simulink model "Target_Control_System"  (R2021b)
settings: Solver=FixedStepDiscrete  StartTime=0.0  StopTime=5  RelTol=1e-3
PreLoadFcn:
  | RTWConfigurationCB('preloadfcn', bdroot);
PostLoadFcn:
  | load('configuration/data_struct.mat');
  | load('configuration/fluxMaps_propMotor.mat');
  | load('configuration/parameterInit_PROP.mat');
  | load('configuration/parameterInit_PUMP.mat');
  | load('configuration/parameterInit_PITCH.mat');
  | load('configuration/parameterInit_TILT.mat');
  | %load('configuration/base_workspace_signal_definition.mat');
  | %load('resolvedatastores_to_baseworkspace_for_faster_simulation.mat');
model workspace (MAT data in the model file):
  SIMULATION_OPTIONS : Simulink.Parameter (value not decoded)
  TARGET_CODE_GEN : Simulink.Parameter (value not decoded)
  TCS_SAMPLE_FREQ_HZ : Simulink.Parameter (value not decoded)
symbols that are objects in the model workspace (value not decoded): TARGET_CODE_GEN, TCS_SAMPLE_FREQ_HZ
undefined symbols (not defined in the file): A_DQ_REF_LPF_INIT__PITCH, A_DQ_REF_LPF_INIT__PROP, A_DQ_REF_LPF_INIT__PUMP, A_DQ_REF_LPF_INIT__TILT, A_OBSERVER_CONFIDENCE_INIT__PITCH, A_OBSERVER_CONFIDENCE_INIT__PROP, A_OBSERVER_CONFIDENCE_INIT__PUMP, A_OBSERVER_CONFIDENCE_INIT__TILT, ACTUATOR_MAX_ANGLE_TRIP__PITCH, ACTUATOR_MIN_ANGLE_TRIP__PITCH, ACTUATOR_POS_SENSOR_INV_DIRECTION__PITCH, ACTUATOR_POS_SENSOR_INV_DIRECTION__TILT, ACTUATOR_POS_SENSOR_OFFSET__PITCH, ACTUATOR_POS_SENSOR_OFFSET__TILT, ADC_scaler1_baseaddr_TILT, ADC_SCALER_FLOAT_TO_FIXPOINT_EXPANSION, ANGLE_ELEC_FROM_SENSOR_OFFSET_INIT__PITCH, ANGLE_ELEC_FROM_SENSOR_OFFSET_INIT__PROP, ANGLE_ELEC_FROM_SENSOR_OFFSET_INIT__PUMP, ANGLE_ELEC_FROM_SENSOR_OFFSET_INIT__TILT, AUTO_CLEAR_FAULTS_ENABLED__PITCH, AUTO_CLEAR_FAULTS_ENABLED__PROP, AUTO_CLEAR_FAULTS_ENABLED__PUMP, AUTO_CLEAR_FAULTS_ENABLED__TILT, AUTO_CLEAR_FAULTS_WAIT_TICKS__PITCH, AUTO_CLEAR_FAULTS_WAIT_TICKS__PROP, AUTO_CLEAR_FAULTS_WAIT_TICKS__PUMP, AUTO_CLEAR_FAULTS_WAIT_TICKS__TILT, AUTO_I_ZERO_IDLE_TICKS__PITCH, AUTO_I_ZERO_IDLE_TICKS__PROP, AUTO_I_ZERO_IDLE_TICKS__PUMP, AUTO_I_ZERO_IDLE_TICKS__TILT, AUTO_I_ZERO_OFFSET_IDC_THRESHOLD__PITCH, AUTO_I_ZERO_OFFSET_IDC_THRESHOLD__PROP, AUTO_I_ZERO_OFFSET_IDC_THRESHOLD__PUMP, AUTO_I_ZERO_OFFSET_IDC_THRESHOLD__TILT, AUTO_I_ZERO_OFFSET_IPH_THRESHOLD__PITCH, AUTO_I_ZERO_OFFSET_IPH_THRESHOLD__PROP, AUTO_I_ZERO_OFFSET_IPH_THRESHOLD__PUMP, AUTO_I_ZERO_OFFSET_IPH_THRESHOLD__TILT, AUTO_SENSORLESS_SWITCHOVER_DISABLE_OMEGA, AUTO_SENSORLESS_SWITCHOVER_ENABLE_OMEGA, AUTO_SENSORLESS_SWITCHOVER_MIN_CONFIDENCE, AUXILIARY_PROTECTION_UNIT_BASEADDR__TILT, blanking_max_error_omega_INIT_PITCH, blanking_max_error_omega_INIT_TILT, blanking_max_error_position_INIT_PITCH, blanking_max_error_position_INIT_TILT, BRUTE_START_I_Q_REF_RAMP_SPEED__PITCH, BRUTE_START_I_Q_REF_RAMP_SPEED__PROP, BRUTE_START_I_Q_REF_RAMP_SPEED__PUMP, BRUTE_START_I_Q_REF_RAMP_SPEED__TILT, CONTROL_LOOP_DT_INIT__PITCH, CONTROL_LOOP_DT_INIT__PROP, CONTROL_LOOP_DT_INIT__PUMP, CONTROL_LOOP_DT_INIT__TILT, CORRECTION_FILTER_SCALE__PITCH, CORRECTION_FILTER_SCALE__PROP, CORRECTION_FILTER_SCALE__PUMP, CORRECTION_FILTER_SCALE__TILT ... (+458)
libraries: simulink x178, Reusables_Lib x24
(part 41 of 47)

== system Target_Control_System/Target_Control_System/MainLoop/tiltMotor_mainLoop/mainTask_tilt/motorTaskMainFastStep(&oTilt)/Mechanical System - Tilt/processSensors(&oPitch)/Input (motor) side sensor/Compute Speed From Sensor ==
  note: // The position sensor also provides speed information (Presently (Jan. 2020), only the resolver does that.)
      | // We just have to scale it:
  note: // We calculate speed by differentiating the position
  note: // Speed is negative, angle jumped from near -pi to near +pi
  note: // Speed is positive, angle jumped from near +pi to near -pi
  note: // multiply with f_control instead for potentially a bit more speed
  fAngleElecFromSensorPrevious : Inport
  fAngleElecFromSensor : Inport  Port=2
  Add1 : Sum  Inputs=+-
  Add2 : Sum  Inputs=-+
  Add3 : Sum
  Constant3 : Constant  Value=2*pi  OutDataTypeStr=single  SampleTime=-1
  Constant4 : Constant  Value=-1.5*pi  OutDataTypeStr=single  SampleTime=-1
  Constant6 : Constant  Value=2*pi  OutDataTypeStr=single  SampleTime=-1
  Constant9 : Constant  Value=1.5*pi  OutDataTypeStr=single  SampleTime=-1
  Data Store Read1 : DataStoreRead  DataStoreName=oTilt  DataStoreElements=oTilt.oMot_.oParam_.fOneOverSensorPolepairs_  IndexOptions=Index vector (dialog)  Indices=1  OutputSizes=1
  Data Store Read2 : DataStoreRead  DataStoreName=oTilt  DataStoreElements=oTilt.oMot_.oIn_.oAdcData_.fMotorSensorSpeed_  IndexOptions=Index vector (dialog)  Indices=1  OutputSizes=1
  Data Store Read3 : DataStoreRead  DataStoreName=oTilt  DataStoreElements=oTilt.oMot_.oParam_.fPolePairs_  IndexOptions=Index vector (dialog)  Indices=1  OutputSizes=1
  Data Store Read4 : DataStoreRead  DataStoreName=oTilt  DataStoreElements=oTilt.oMot_.oParam_.uiUseOmegaEReportedBySensor_  IndexOptions=Index vector (dialog)  Indices=1  OutputSizes=1
  Data Store Read5 : DataStoreRead  DataStoreName=oTilt  DataStoreElements=oTilt.oIsr_.oParam_.fControlLoopDt_  IndexOptions=Index vector (dialog)  Indices=1  OutputSizes=1
  Data Store Write41 : DataStoreWrite  DataStoreName=oTilt  DataStoreElements=oTilt.oMot_.oState_.oPosSensor_.fAngleElecFromSensorPrevious_  IndexOptions=Index vector (dialog)  Indices=1  OutputSizes=1
  Divide1 : Product  Inputs=***
  Divide2 : Product  Inputs=*/
  GreaterThan1 : RelationalOperator  Operator=>  OutDataTypeStr=boolean  RndMeth=Simplest
  Less Than1 : RelationalOperator  Operator=<  OutDataTypeStr=boolean  RndMeth=Simplest
  Switch2 : Switch  Criteria=u2 > Threshold
  Switch3 : Switch  Criteria=u2 > Threshold
  Switch4 : Switch  Criteria=u2 > Threshold
  softwareIirFilterStep()1 : Subsystem
  fOmegaEFromSensor : Outport
  AngleCurrent : Outport  Port=2
  wires:
  Add1/1 -> GreaterThan1/1, Add2/2, Switch3/3  "fAngleDifference"
  Switch4/1 -> Divide2/1
  Less Than1/1 -> Switch4/2
  Data Store Read5/1 -> Divide2/2
  Data Store Read1/1 -> Divide1/3
  Divide1/1 -> Switch2/1
  Add2/1 -> Switch3/1
  GreaterThan1/1 -> Switch3/2
  softwareIirFilterStep()1/1(fFilterOutput) -> Switch2/3
  Constant3/1 -> Add2/1
  Divide2/1 -> softwareIirFilterStep()1/1(fNewInput)  "fOmegaVeryRaw"
  Data Store Read3/1 -> Divide1/2
  Data Store Read4/1 -> Switch2/2
  Constant4/1 -> Less Than1/2
  Constant6/1 -> Add3/1
  fAngleElecFromSensor/1 -> Add1/1, Data Store Write41/1, AngleCurrent/1
  Data Store Read2/1 -> Divide1/1
  fAngleElecFromSensorPrevious/1 -> Add1/2
  Switch2/1 -> fOmegaEFromSensor/1
  Add3/1 -> Switch4/1
  Switch3/1 -> Switch4/3, Less Than1/1, Add3/2
  Constant9/1 -> GreaterThan1/2

== system Target_Control_System/Target_Control_System/MainLoop/tiltMotor_mainLoop/mainTask_tilt/motorTaskMainFastStep(&oTilt)/Mechanical System - Tilt/processSensors(&oPitch)/Input (motor) side sensor/PosSensorProcess_altImplementations ==
  note: // --- Compute speed from sensor ---
  note: // --- Compute speed by differentiation of position ---
  Constant10 : Constant  Commented=on  Value=-pi  OutDataTypeStr=single
  Constant7 : Constant  Commented=on  OutDataTypeStr=single
  Constant8 : Constant  Commented=on  Value=pi  OutDataTypeStr=single
  Constant9 : Constant  Commented=on  OutDataTypeStr=single
  Data Store Read{4,13,23..24} (4 alike) : DataStoreRead  Commented=on  DataStoreName=oTilt  DataStoreElements=oTilt.oMot_.oState_.oPosSensor_.fAngleElecFromSensor_  IndexOptions=Index vector (dialog)  Indices=1  OutputSizes=1
  Data Store Read20 : DataStoreRead  Commented=on  DataStoreName=oTilt  DataStoreElements=oTilt.oMot_.oParam_.uiUseOmegaEReportedBySensor_  IndexOptions=Index vector (dialog)  Indices=1  OutputSizes=1
  Data Store Read21 : DataStoreRead  Commented=on  DataStoreName=oTilt  DataStoreElements=oTilt.oMot_.oIn_.oAdcData_.fMotorSensorSpeed_  IndexOptions=Index vector (dialog)  Indices=1  OutputSizes=1
  Data Store Write12 : DataStoreWrite  Commented=on  DataStoreName=oTilt  DataStoreElements=oTilt.oMot_.oState_.oPosSensor_.fOmegaEFromSensor_  IndexOptions=Index vector (dialog)  Indices=1  OutputSizes=1
  Data Store Write13 : DataStoreWrite  Commented=on  DataStoreName=oTilt  DataStoreElements=oTilt.oMot_.oState_.oPosSensor_.fAngleElecFromSensorPrevious_  IndexOptions=Index vector (dialog)  Indices=1  OutputSizes=1
  Data Store Write14 : DataStoreWrite  Commented=on  DataStoreName=oTilt  DataStoreElements=oTilt.oMot_.oState_.oPosSensor_.fOmegaEFromSensor_  IndexOptions=Index vector (dialog)  Indices=1  OutputSizes=1
  Data Store Write15 : DataStoreWrite  Commented=on  DataStoreName=oTilt  DataStoreElements=oTilt.oMot_.oState_.oPosSensor_.fAngleElecFromSensorPrevious_  IndexOptions=Index vector (dialog)  Indices=1  OutputSizes=1
  Display : Display  Commented=on
  Display1 : Display  Commented=on
  GreaterThan2 : RelationalOperator  Commented=on  Operator=>  OutDataTypeStr=boolean  RndMeth=Simplest
  GreaterThan3 : RelationalOperator  Commented=on  Operator=<  OutDataTypeStr=boolean  RndMeth=Simplest
  If Action Subsystem : Subsystem  Commented=on  TreatAsAtomicUnit=on
  If Action Subsystem1 : Subsystem  Commented=on  TreatAsAtomicUnit=on
  If1 : If  Commented=on
  Triggered Subsystem : Subsystem  Commented=on  TreatAsAtomicUnit=on
  Triggered Subsystem1 : Subsystem  Commented=on  TreatAsAtomicUnit=on
  While Iterator Subsystem : Subsystem  Commented=on  TreatAsAtomicUnit=on
  While Iterator Subsystem1 : Subsystem  Commented=on  TreatAsAtomicUnit=on
  wires:
  Constant8/1 -> GreaterThan2/2
  Data Store Read23/1 -> Triggered Subsystem/1(In1)
  Constant9/1 -> While Iterator Subsystem1/2(IC)
  If1/1 -> If Action Subsystem/Action
  Triggered Subsystem1/1(Out1) -> Data Store Write15/1
  While Iterator Subsystem1/1(Out1) -> Display1/1
  Data Store Read20/1 -> If1/1
  Data Store Read21/1 -> If Action Subsystem/1(In1)
  Constant7/1 -> While Iterator Subsystem/2(IC)
  If Action Subsystem/1(Out1) -> Triggered Subsystem1/Trigger, Data Store Write14/1
  Constant10/1 -> GreaterThan3/2
  Triggered Subsystem/1(Out1) -> Data Store Write13/1
  If Action Subsystem1/1(fFilterOutput) -> Data Store Write12/1, Triggered Subsystem/Trigger
  While Iterator Subsystem/1(Out1) -> Display/1
  If1/2 -> If Action Subsystem1/Action
  Data Store Read24/1 -> Triggered Subsystem1/1(In1)
  Data Store Read13/1 -> GreaterThan2/1
  GreaterThan2/1 -> While Iterator Subsystem/1(In1)
  Data Store Read4/1 -> GreaterThan3/1
  GreaterThan3/1 -> While Iterator Subsystem1/1(In1)

== system Target_Control_System/Target_Control_System/MainLoop/tiltMotor_mainLoop/mainTask_tilt/motorTaskMainFastStep(&oTilt)/Mechanical System - Tilt/processSensors(&oPitch)/Input (motor) side sensor/Stuck Sensor Detection ==
  note: / We want to detect bitwise identical values, so a hard equal comparison on two floats is exactly intended
  fAngleElecFromSensor : Inport
  NumOfIdenticalValues : Inport  Port=2
  fAngleElecFromSensorPrevious : Inport  Port=3
  Add14 : Sum
  Constant12 : Constant  Value=0  OutDataTypeStr=int32  SampleTime=-1
  Constant13 : Constant  OutDataTypeStr=int32  SampleTime=-1
  Data Store Write1 : DataStoreWrite  DataStoreName=oTilt  DataStoreElements=oTilt.oMot_.oState_.oPosSensor_.iAngleElecFromSensorNumOfIdenticalValues_  IndexOptions=Index vector (dialog)  Indices=1  OutputSizes=1
  GreaterThan4 : RelationalOperator  Operator===  OutDataTypeStr=boolean  RndMeth=Simplest
  Switch13 : Switch  Criteria=u2 > Threshold
  wires:
  NumOfIdenticalValues/1 -> Add14/1
  Constant13/1 -> Add14/2
  fAngleElecFromSensorPrevious/1 -> GreaterThan4/2
  fAngleElecFromSensor/1 -> GreaterThan4/1
  Add14/1 -> Switch13/1
  Constant12/1 -> Switch13/3
  Switch13/1 -> Data Store Write1/1
  GreaterThan4/1 -> Switch13/2

== system Target_Control_System/Target_Control_System/MainLoop/tiltMotor_mainLoop/mainTask_tilt/motorTaskMainFastStep(&oTilt)/Mechanical System - Tilt/processSensors(&oPitch)/Input (motor) side sensor/updateGbxOutput ==
  fNewInputAngle : Inport
  AND2 : Logic  AllPortsSameDT=off  OutDataTypeStr=boolean
  AND3 : Logic  AllPortsSameDT=off  OutDataTypeStr=boolean
  Add3 : Sum
  Add4 : Sum  Inputs=-+
  Add5 : Sum  Inputs=+++
  Constant10 : Constant  Value=-pi/2  OutDataTypeStr=single  SampleTime=-1
  Constant11 : Constant  Value=2*pi  OutDataTypeStr=single  SampleTime=-1
  Constant6 : Constant  Value=pi/2  OutDataTypeStr=single  SampleTime=-1
  Constant7 : Constant  Value=-pi/2  OutDataTypeStr=single  SampleTime=-1
  Constant8 : Constant  OutDataTypeStr=single  SampleTime=-1
  Constant9 : Constant  Value=pi/2  OutDataTypeStr=single  SampleTime=-1
  Data Store Read4 : DataStoreRead  DataStoreName=oTilt  DataStoreElements=oTilt.oMot_.oState_.oPosSensor_.oGbx_.iFullInputRevolutions_  IndexOptions=Index vector (dialog)  Indices=1  OutputSizes=1
  Data Store Read5 : DataStoreRead  DataStoreName=oTilt  DataStoreElements=oTilt.oMot_.oState_.oPosSensor_.oGbx_.fGbxRatio_  IndexOptions=Index vector (dialog)  Indices=1  OutputSizes=1
  Data Store Read6 : DataStoreRead  DataStoreName=oTilt  DataStoreElements=oTilt.oMot_.oState_.oPosSensor_.oGbx_.fOutputOffset_  IndexOptions=Index vector (dialog)  Indices=1  OutputSizes=1
  Data Store Read7 : DataStoreRead  DataStoreName=oTilt  DataStoreElements=oTilt.oMot_.oState_.oPosSensor_.oGbx_.fPreviousInputAngle_  IndexOptions=Index vector (dialog)  Indices=1  OutputSizes=1
  Data Store Write1 : DataStoreWrite  DataStoreName=oTilt  DataStoreElements=oTilt.oMot_.oState_.oPosSensor_.oGbx_.iFullInputRevolutions_  IndexOptions=Index vector (dialog)  Indices=1  OutputSizes=1
  Divide2 : Product  Inputs=**/
  Divide3 : Product  Inputs=/*
  GreaterThan2 : RelationalOperator  Operator=>  OutDataTypeStr=boolean  RndMeth=Simplest
  GreaterThan3 : RelationalOperator  Operator=>  OutDataTypeStr=boolean  RndMeth=Simplest
  Less Than2 : RelationalOperator  Operator=<  OutDataTypeStr=boolean  RndMeth=Simplest
  Less Than3 : RelationalOperator  Operator=<  OutDataTypeStr=boolean  RndMeth=Simplest
  Switch2 : Switch  Criteria=u2 > Threshold
  Switch3 : Switch  Criteria=u2 > Threshold  OutDataTypeStr=int32
  updateAngles : Subsystem
  fCurrentOutputAngle : Outport
  wires:
  Less Than3/1 -> AND3/1
  Data Store Read4/1 -> Switch2/3, Add4/2, Add3/2
  Data Store Read7/1 -> GreaterThan2/1, Less Than3/1
  Add4/1 -> Switch3/1
  GreaterThan2/1 -> AND2/2
  Data Store Read6/1 -> Add5/3
  Switch2/1 -> Switch3/3
  fNewInputAngle/1 -> Less Than2/1, GreaterThan3/1, Divide3/2, updateAngles/2(fNewInputAngle)
  Divide3/1 -> Add5/2
  Add3/1 -> Switch2/1
  Data Store Read5/1 -> Divide2/3, Divide3/1
  Constant11/1 -> Divide2/2
  Constant6/1 -> GreaterThan2/2
  Constant7/1 -> Less Than2/2
  Divide2/1 -> Add5/1
  AND2/1 -> Switch2/2
  AND3/1 -> Switch3/2
  Constant8/1 -> Add3/1, Add4/1
  Constant10/1 -> Less Than3/2
  GreaterThan3/1 -> AND3/2
  Switch3/1 -> Divide2/1, Data Store Write1/1
  Less Than2/1 -> AND2/1
  Add5/1 -> updateAngles/1(fCurrentOutputAngle), fCurrentOutputAngle/1
  Constant9/1 -> GreaterThan3/2

== system Target_Control_System/Target_Control_System/MainLoop/tiltMotor_mainLoop/mainTask_tilt/motorTaskMainFastStep(&oTilt)/Software Overcurrent Protection - Tilt/checkForHwOvercurrents(&oTilt)/gateDriverStatus/DoNotIncludeCustomCode ==
  Constant : Constant  Value=0  OutDataTypeStr=uint32
  Data Store Write : DataStoreWrite  DataStoreName=oTilt  DataStoreElements=oTilt.oMot_.oOut_.uiGateDriverStatus_  IndexOptions=Index vector (dialog)  Indices=1  OutputSizes=1
  Data Store Write1 : DataStoreWrite  DataStoreName=mdl_tilt_uiFlags  IndexOptions=Index vector (dialog)  Indices=1  OutputSizes=1
  Data Store Write2 : DataStoreWrite  DataStoreName=mdl_tilt_uiAPUFlags  IndexOptions=Index vector (dialog)  Indices=1  OutputSizes=1
  wires:
  Constant/1 -> Data Store Write/1, Data Store Write1/1, Data Store Write2/1

== system Target_Control_System/Target_Control_System/MainLoop/tiltMotor_mainLoop/mainTask_tilt/motorTaskMainFastStep(&oTilt)/Software Overcurrent Protection - Tilt/checkForHwOvercurrents(&oTilt)/gateDriverStatus/IncludeCustomCode ==
  System Update : Subsystem  mask(System Update){ShowInLibBrowser=0}
      mask prompts: ShowInLibBrowser "Simulink:masks:CustCodeMaskParam1_MP"
      settings: CopyFcn=cccopyfcn(gcb)  OpenFcn=ccopenfcn('System Update Function')
      mask Help: eval('feval(''rtwprivate'',''rtwhelpview'',''rtw_sys_update_block'')');
      mask DialogControl ShowInLibBrowser Prompt: Mask Parameter 1:
      mask Display: disp('System\nUpdate');

== system Target_Control_System/Target_Control_System/Simulation Controls/Simulation Data Store Initialization/setupPwm(&oTilt)/setPwmFrequencyApplication()_tilt/setPwmFrequency()_tilt/updateServoObserver()_tilt/softwareIirFilterInitialize()/computeCoefficientsButter() ==
  fCutoffFrequencyHz : Inport  OutDataTypeStr=single
  dSampleFrequencyHz : Inport  Port=2  OutDataTypeStr=single
  Add : Sum  Inputs=+++  OutDataTypeStr=double
  Add1 : Sum  Inputs=-+
  Add2 : Sum  Inputs=+-+  OutDataTypeStr=double
  Constant : Constant  Value=0.0008  OutDataTypeStr=single
  Constant1 : Constant  Value=0.45  OutDataTypeStr=single
  Constant{5,7,9..10} (4 alike) : Constant
  Constant2 : Constant  Value=pi  OutDataTypeStr=double
  Constant3 : Constant  OutDataTypeStr=double
  Constant4 : Constant  Value=sqrt(2)  OutDataTypeStr=double
  Constant6 : Constant  OutDataTypeStr=double
  Constant8 : Constant  Value=2
  Data Type Conversion : DataTypeConversion  OutDataTypeStr=double
  Divide : Product  Inputs=**  OutDataTypeStr=single
  Divide1 : Product  Inputs=**  OutDataTypeStr=single
  Divide{3,5..6,8,10..11} (6 alike) : Product  Inputs=**  OutDataTypeStr=double
  Divide2 : Product  Inputs=*/  OutDataTypeStr=double
  Divide4 : Product  Inputs=*/  OutDataTypeStr=double
  Divide7 : Product  Inputs=*/  OutDataTypeStr=double
  Divide9 : Product  Inputs=***  OutDataTypeStr=double
  Gain : Gain  Gain=2  OutDataTypeStr=double
  Gain1 : Gain  Gain=-1  OutDataTypeStr=double
  Gain2 : Gain  Gain=-1  OutDataTypeStr=double
  Gain3 : Gain  Gain=-1  OutDataTypeStr=double
  Mux : Mux  Inputs=6
  Saturation Dynamic : simulink/Discontinuities/Saturation Dynamic  OutMin=[]  OutMax=[]  OutDataTypeStr=Inherit: Same as second input  OutDataType=fixdt(1, 16)  OutScaling=2^-10  DoSatur=off
  Tan : Trigonometry  Operator=tan
  dpOutArray : Outport
  fFreq3db : Outport  Port=2
  wires:
  Data Type Conversion/1 -> Divide2/1
  Constant10/1 -> Mux/4
  [dA2] -> Gain3/1
  Gain3/1 -> Mux/6
  [dA1] -> Gain2/1
  Gain2/1 -> Mux/5
  [dB2] -> Mux/3
  [dB1] -> Mux/2
  [dB0] -> Mux/1
  Divide11/1 -> [dA2]
  Gain1/1 -> Divide11/2
  Add2/1 -> Gain1/1
  Constant9/1 -> Add2/3
  Divide10/1 -> Add2/2
  [kdQ] -> Divide10/2
  Constant7/1 -> Add1/1
  Divide8/1 -> Add1/2, Add2/1
  Divide9/1 -> [dA1]
  Constant8/1 -> Divide9/3
  Add1/1 -> Divide9/2
  [kdIta] -> Divide8/1, Divide8/2, Divide10/1
  Gain/1 -> [dB1]
  Divide7/1 -> [dB0], Gain/1, [dB2], Divide9/1, Divide11/1
  Add/1 -> Divide7/2
  Constant6/1 -> Divide7/1
  Constant5/1 -> Add/3
  Divide5/1 -> Add/2
  Divide6/1 -> Add/1
  [kdQ] -> Divide5/2
  [kdIta] -> Divide5/1, Divide6/1, Divide6/2
  Mux/1 -> dpOutArray/1
  Constant4/1 -> [kdQ]
  Divide4/1 -> [kdIta]
  Constant3/1 -> Divide4/1
  Tan/1 -> Divide4/2
  Divide3/1 -> Tan/1
  Constant2/1 -> Divide3/2
  Divide2/1 -> Divide3/1  "dFf"
  Constant/1 -> Divide/2
  Saturation Dynamic/1 -> fFreq3db/1, Data Type Conversion/1  "fCutoffFrequencyHz"
  Divide1/1 -> Saturation Dynamic/1
  dSampleFrequencyHz/1 -> Divide1/2, Divide2/2, Divide/1
  Constant1/1 -> Divide1/1
  Divide/1 -> Saturation Dynamic/3
  fCutoffFrequencyHz/1 -> Saturation Dynamic/2

== system Target_Control_System/Target_Control_System/Simulation Controls/Simulation Data Store Initialization/setupPwm()/setPwmFrequencyApplication()_pitch/setPwmFrequency()_pitch/updateServoObserver()_pitch/softwareIirFilterInitialize()/computeCoefficientsButter() ==
  fCutoffFrequencyHz : Inport  OutDataTypeStr=single
  dSampleFrequencyHz : Inport  Port=2  OutDataTypeStr=single
  Add : Sum  Inputs=+++  OutDataTypeStr=double
  Add1 : Sum  Inputs=-+
  Add2 : Sum  Inputs=+-+  OutDataTypeStr=double
  Constant : Constant  Value=0.0008  OutDataTypeStr=single
  Constant1 : Constant  Value=0.45  OutDataTypeStr=single
  Constant{5,7,9..10} (4 alike) : Constant
  Constant2 : Constant  Value=pi  OutDataTypeStr=double
  Constant3 : Constant  OutDataTypeStr=double
  Constant4 : Constant  Value=sqrt(2)  OutDataTypeStr=double
  Constant6 : Constant  OutDataTypeStr=double
  Constant8 : Constant  Value=2
  Data Type Conversion : DataTypeConversion  OutDataTypeStr=double
  Divide : Product  Inputs=**  OutDataTypeStr=single
  Divide1 : Product  Inputs=**  OutDataTypeStr=single
  Divide{3,5..6,8,10..11} (6 alike) : Product  Inputs=**  OutDataTypeStr=double
  Divide2 : Product  Inputs=*/  OutDataTypeStr=double
  Divide4 : Product  Inputs=*/  OutDataTypeStr=double
  Divide7 : Product  Inputs=*/  OutDataTypeStr=double
  Divide9 : Product  Inputs=***  OutDataTypeStr=double
  Gain : Gain  Gain=2  OutDataTypeStr=double
  Gain1 : Gain  Gain=-1  OutDataTypeStr=double
  Gain2 : Gain  Gain=-1  OutDataTypeStr=double
  Gain3 : Gain  Gain=-1  OutDataTypeStr=double
  Mux : Mux  Inputs=6
  Saturation Dynamic : simulink/Discontinuities/Saturation Dynamic  OutMin=[]  OutMax=[]  OutDataTypeStr=Inherit: Same as second input  OutDataType=fixdt(1, 16)  OutScaling=2^-10  DoSatur=off
  Tan : Trigonometry  Operator=tan
  dpOutArray : Outport
  fFreq3db : Outport  Port=2
  wires:
  Data Type Conversion/1 -> Divide2/1
  Constant10/1 -> Mux/4
  [dA2] -> Gain3/1
  Gain3/1 -> Mux/6
  [dA1] -> Gain2/1
  Gain2/1 -> Mux/5
  [dB2] -> Mux/3
  [dB1] -> Mux/2
  [dB0] -> Mux/1
  Divide11/1 -> [dA2]
  Gain1/1 -> Divide11/2
  Add2/1 -> Gain1/1
  Constant9/1 -> Add2/3
  Divide10/1 -> Add2/2
  [kdQ] -> Divide10/2
  Constant7/1 -> Add1/1
  Divide8/1 -> Add1/2, Add2/1
  Divide9/1 -> [dA1]
  Constant8/1 -> Divide9/3
  Add1/1 -> Divide9/2
  [kdIta] -> Divide8/1, Divide8/2, Divide10/1
  Gain/1 -> [dB1]
  Divide7/1 -> [dB0], Gain/1, [dB2], Divide9/1, Divide11/1
  Add/1 -> Divide7/2
  Constant6/1 -> Divide7/1
  Constant5/1 -> Add/3
  Divide5/1 -> Add/2
  Divide6/1 -> Add/1
  [kdQ] -> Divide5/2
  [kdIta] -> Divide5/1, Divide6/1, Divide6/2
  Mux/1 -> dpOutArray/1
  Constant4/1 -> [kdQ]
  Divide4/1 -> [kdIta]
  Constant3/1 -> Divide4/1
  Tan/1 -> Divide4/2
  Divide3/1 -> Tan/1
  Constant2/1 -> Divide3/2
  Divide2/1 -> Divide3/1  "dFf"
  Constant/1 -> Divide/2
  Saturation Dynamic/1 -> fFreq3db/1, Data Type Conversion/1  "fCutoffFrequencyHz"
  Divide1/1 -> Saturation Dynamic/1
  dSampleFrequencyHz/1 -> Divide1/2, Divide2/2, Divide/1
  Constant1/1 -> Divide1/1
  Divide/1 -> Saturation Dynamic/3
  fCutoffFrequencyHz/1 -> Saturation Dynamic/2

== system Target_Control_System/Target_Control_System/MainLoop/pitchMotor_mainLoop/Decimation gate for 200 Hz Pitch/Function-Call Subsystem/Position control checks/Position control mode/Check fighting controllers/Enabled Subsystem/Enabled Subsystem ==
  note: This is the slave inverter
  Enable : EnablePort
  Chart : Stateflow chart  TreatAsAtomicUnit=on

== system Target_Control_System/Target_Control_System/MainLoop/pitchMotor_mainLoop/Decimation gate for 200 Hz Pitch/Function-Call Subsystem/Position control checks/Position control mode/checkSensorLimits(&oPitch)/Check broken sensor/All other sensor types ==
  note: All other sensors have a similar interface
  Enable : EnablePort
  Chart : Stateflow chart  TreatAsAtomicUnit=on

== system Target_Control_System/Target_Control_System/MainLoop/pitchMotor_mainLoop/Decimation gate for 200 Hz Pitch/Function-Call Subsystem/Position control checks/Position control mode/checkSensorLimits(&oPitch)/Check broken sensor/Resolver ==
  note: This one is somewhat special.
      | The fault code is the 8 bit word coming from the AD2S1210 resolver interface.
      | Some bits are warnigs, some are errors.
      | On ideal hardware the reported code is zero, but we're not quite there yet.
      | From the data sheet:
      |     Table 26. Fault Register Bit Descriptions
      |     Bit  Description
      |     D7   Sine/cosine inputs clipped
      |     D6   Sine/cosine inputs below LOS threshold
      |     D5   Sine/cosine inputs exceed DOS overrange threshold
      |     D4   Sine/cosine inputs exceed DOS mismatch threshold
      |     D3   Tracking error exceeds LOT threshold
      |     D2   Velocity exceeds maximum tracking rate
      |     D1   Phase error exceeds phase lock range
      |     D0   Configuration parity error
      | Understanding in November 2019:
      |     D0-D3 are generally 'true' errors (if set, the result is garbage)
      |     D4-D7 are generally warnings. (often when set, the angle result is actually still valid)
  Enable : EnablePort
  Chart : Stateflow chart  TreatAsAtomicUnit=on

== system Target_Control_System/Target_Control_System/MainLoop/pitchMotor_mainLoop/Decimation gate for 200 Hz Pitch/Function-Call Subsystem/Position control checks/Position control mode/checkSensorLimits(&oPitch)/Check delta input-output/Enabled Subsystem ==
  Enable : EnablePort
  Chart : Stateflow chart  TreatAsAtomicUnit=on

== system Target_Control_System/Target_Control_System/MainLoop/pitchMotor_mainLoop/Decimation gate for 200 Hz Pitch/Function-Call Subsystem/Position control checks/Position control mode/checkSensorLimits(&oPitch)/Check for stuck sensor/Enabled Subsystem ==
  Enable : EnablePort
  Chart : Stateflow chart  TreatAsAtomicUnit=on

== system Target_Control_System/Target_Control_System/MainLoop/pitchMotor_mainLoop/Decimation gate for 200 Hz Pitch/Function-Call Subsystem/Position control checks/Position control mode/checkSensorLimits(&oPitch)/Read sensor flags/nonresolverSensorCodes ==
  Enable : EnablePort
  ModelSource : Subsystem  Variant=on

== system Target_Control_System/Target_Control_System/MainLoop/pitchMotor_mainLoop/Decimation gate for 200 Hz Pitch/Function-Call Subsystem/Position control checks/Position control mode/checkSensorLimits(&oPitch)/Read sensor flags/resolverSensorCodes ==
  Enable : EnablePort
  ModelSource : Subsystem  Variant=on

== system Target_Control_System/Target_Control_System/MainLoop/pitchMotor_mainLoop/mainTask_pitch/motorTaskMainFastStep()/Automatic switching to sensorless - Pitch/Automatic switching to sensorless/Switch to sensored /Switch to sensored/Angle To +-pi ==
  Angle In : Inport
  Add4 : Sum  Inputs=-+
  Add5 : Sum
  Equal4 : RelationalOperator  Operator=>  OutDataTypeStr=boolean  RndMeth=Simplest
  Equal6 : RelationalOperator  Operator=<  OutDataTypeStr=boolean  RndMeth=Simplest
  Pi5 : Constant  Value=pi  OutDataTypeStr=single  SampleTime=-1
  Pi6 : Constant  Value=2*pi  OutDataTypeStr=single  SampleTime=-1
  Pi7 : Constant  Value=-pi  OutDataTypeStr=single  SampleTime=-1
  Pi9 : Constant  Value=2*pi  OutDataTypeStr=single  SampleTime=-1
  Switch : Switch  Criteria=u2 > Threshold
  Switch4 : Switch  Criteria=u2 > Threshold
  Angle Out : Outport
  wires:
  Switch/1 -> Equal6/1, Add5/2, Switch4/3
  Pi7/1 -> Equal6/2
  Add4/1 -> Switch/1
  Pi9/1 -> Add5/1
  Pi5/1 -> Equal4/2
  Equal4/1 -> Switch/2
  Switch4/1 -> Angle Out/1
  Angle In/1 -> Equal4/1, Add4/2, Switch/3
  Add5/1 -> Switch4/1
  Equal6/1 -> Switch4/2
  Pi6/1 -> Add4/1

== system Target_Control_System/Target_Control_System/MainLoop/pitchMotor_mainLoop/mainTask_pitch/motorTaskMainFastStep()/Automatic switching to sensorless - Pitch/Automatic switching to sensorless/Switch to sensorless?/Switch to sensorless/Angle To +-pi ==
  Angle In : Inport
  Add4 : Sum  Inputs=-+
  Add5 : Sum
  Equal4 : RelationalOperator  Operator=>  OutDataTypeStr=boolean  RndMeth=Simplest
  Equal6 : RelationalOperator  Operator=<  OutDataTypeStr=boolean  RndMeth=Simplest
  Pi5 : Constant  Value=pi  OutDataTypeStr=single  SampleTime=-1
  Pi6 : Constant  Value=2*pi  OutDataTypeStr=single  SampleTime=-1
  Pi7 : Constant  Value=-pi  OutDataTypeStr=single  SampleTime=-1
  Pi9 : Constant  Value=2*pi  OutDataTypeStr=single  SampleTime=-1
  Switch : Switch  Criteria=u2 > Threshold
  Switch4 : Switch  Criteria=u2 > Threshold
  Angle Out : Outport
  wires:
  Switch/1 -> Equal6/1, Add5/2, Switch4/3
  Pi7/1 -> Equal6/2
  Add4/1 -> Switch/1
  Pi9/1 -> Add5/1
  Pi5/1 -> Equal4/2
  Equal4/1 -> Switch/2
  Switch4/1 -> Angle Out/1
  Angle In/1 -> Equal4/1, Add4/2, Switch/3
  Add5/1 -> Switch4/1
  Equal6/1 -> Switch4/2
  Pi6/1 -> Add4/1

== system Target_Control_System/Target_Control_System/MainLoop/pitchMotor_mainLoop/mainTask_pitch/motorTaskMainFastStep()/Mechanical System - Pitch/processSensors(&oPitch)/Input (motor) side sensor/ /angleClip (+-pi) ==
  Angle_In : Inport
  Add1 : Sum  Inputs=-+
  Add12 : Sum  Inputs=-+
  Add2 : Sum
  Add3 : Sum
  Equal1 : RelationalOperator  Operator=>  OutDataTypeStr=boolean  RndMeth=Simplest
  Equal2 : RelationalOperator  Operator=<  OutDataTypeStr=boolean  RndMeth=Simplest
  Equal3 : RelationalOperator  Operator=<  OutDataTypeStr=boolean  RndMeth=Simplest
  Equal5 : RelationalOperator  Operator=>  OutDataTypeStr=boolean  RndMeth=Simplest
  Pi : Constant  Value=pi  OutDataTypeStr=single  SampleTime=-1
  Pi1 : Constant  Value=2*pi  OutDataTypeStr=single  SampleTime=-1
  Pi2 : Constant  Value=-pi  OutDataTypeStr=single  SampleTime=-1
  Pi3 : Constant  Value=2*pi  OutDataTypeStr=single  SampleTime=-1
  Pi4 : Constant  Value=-pi  OutDataTypeStr=single  SampleTime=-1
  Pi8 : Constant  Value=pi  OutDataTypeStr=single  SampleTime=-1
  Switch{1..3,5} (4 alike) : Switch  Criteria=u2 > Threshold  Threshold=0.5
  Angle_Out : Outport
  wires:
  Switch3/1 -> Switch2/1
  Equal2/1 -> Switch3/2
  Switch5/1 -> Switch2/3, Add3/2, Equal3/1
  Add2/1 -> Switch3/1
  Pi3/1 -> Add3/1, Add2/1
  Add3/1 -> Switch3/3, Equal2/1, Add2/2
  Pi4/1 -> Equal2/2
  Switch2/1 -> Angle_Out/1
  Equal3/1 -> Switch2/2
  Pi2/1 -> Equal3/2
  Switch1/1 -> Switch5/1
  Add1/1 -> Switch1/1
  Equal5/1 -> Switch1/2
  Pi8/1 -> Equal5/2
  Add12/1 -> Equal5/1, Add1/2, Switch1/3
  Pi/1 -> Equal1/2
  Equal1/1 -> Switch5/2
  Angle_In/1 -> Add12/2, Equal1/1, Switch5/3
  Pi1/1 -> Add12/1, Add1/1

== system Target_Control_System/Target_Control_System/MainLoop/pitchMotor_mainLoop/mainTask_pitch/motorTaskMainFastStep()/Mechanical System - Pitch/processSensors(&oPitch)/Input (motor) side sensor/Compute Speed From Sensor/softwareIirFilterStep() ==
  fNewInput : Inport
  Add : Sum  Inputs=+++--
  Constant : Constant  Value=0  OutDataTypeStr=single  SampleTime=-1
  Constant1 : Constant  Value=0  OutDataTypeStr=single  SampleTime=-1
  Data Store Read : DataStoreRead  DataStoreName=oPitch  DataStoreElements=oPitch.oMot_.oState_.oPosSensor_.oInputSensorSpeedFilter_.afPreviousInputs_.h0  IndexOptions=Index vector (dialog)  Indices=1  OutputSizes=1
  Data Store Read1 : DataStoreRead  DataStoreName=oPitch  DataStoreElements=oPitch.oMot_.oState_.oPosSensor_.oInputSensorSpeedFilter_.afPreviousInputs_.h1  IndexOptions=Index vector (dialog)  Indices=1  OutputSizes=1
  Data Store Read2 : DataStoreRead  DataStoreName=oPitch  DataStoreElements=oPitch.oMot_.oState_.oPosSensor_.oInputSensorSpeedFilter_.afConstantsB_.h0  IndexOptions=Index vector (dialog)  Indices=1  OutputSizes=1
  Data Store Read3 : DataStoreRead  DataStoreName=oPitch  DataStoreElements=oPitch.oMot_.oState_.oPosSensor_.oInputSensorSpeedFilter_.afConstantsB_.h1  IndexOptions=Index vector (dialog)  Indices=1  OutputSizes=1
  Data Store Read4 : DataStoreRead  DataStoreName=oPitch  DataStoreElements=oPitch.oMot_.oState_.oPosSensor_.oInputSensorSpeedFilter_.afConstantsB_.h2  IndexOptions=Index vector (dialog)  Indices=1  OutputSizes=1
  Data Store Read5 : DataStoreRead  DataStoreName=oPitch  DataStoreElements=oPitch.oMot_.oState_.oPosSensor_.oInputSensorSpeedFilter_.afConstantsA_.h1  IndexOptions=Index vector (dialog)  Indices=1  OutputSizes=1
  Data Store Read6 : DataStoreRead  DataStoreName=oPitch  DataStoreElements=oPitch.oMot_.oState_.oPosSensor_.oInputSensorSpeedFilter_.afPreviousOutputs_.h0  IndexOptions=Index vector (dialog)  Indices=1  OutputSizes=1
  Data Store Read7 : DataStoreRead  DataStoreName=oPitch  DataStoreElements=oPitch.oMot_.oState_.oPosSensor_.oInputSensorSpeedFilter_.afConstantsA_.h2  IndexOptions=Index vector (dialog)  Indices=1  OutputSizes=1
  Data Store Read8 : DataStoreRead  DataStoreName=oPitch  DataStoreElements=oPitch.oMot_.oState_.oPosSensor_.oInputSensorSpeedFilter_.afPreviousOutputs_.h1  IndexOptions=Index vector (dialog)  Indices=1  OutputSizes=1
  Data Store Read9 : DataStoreRead  DataStoreName=oPitch  DataStoreElements=oPitch.oMot_.oState_.oPosSensor_.oInputSensorSpeedFilter_.afConstantsA_.h0  IndexOptions=Index vector (dialog)  Indices=1  OutputSizes=1
  Data Store Write41 : DataStoreWrite  DataStoreName=oPitch  DataStoreElements=oPitch.oMot_.oState_.oPosSensor_.oInputSensorSpeedFilter_.fFilterOutput_  IndexOptions=Index vector (dialog)  Indices=1  OutputSizes=1
  Divide{,1..5} (6 alike) : Product  Inputs=**
  IsInf : RelationalOperator  Operator=isInf  OutDataTypeStr=boolean  RndMeth=Simplest
  IsInf1 : RelationalOperator  Operator=isInf  OutDataTypeStr=boolean  RndMeth=Simplest
  IsNaN : RelationalOperator  Operator=isNaN  OutDataTypeStr=boolean  RndMeth=Simplest
  IsNaN1 : RelationalOperator  Operator=isNaN  OutDataTypeStr=boolean  RndMeth=Simplest
  Switch{,1..3} (4 alike) : Switch  Criteria=u2 > Threshold
  prepare for next round : Subsystem
  fFilterOutput : Outport
  wires:
  Divide5/1 -> fFilterOutput/1, Data Store Write41/1
  Data Store Read9/1 -> Divide5/1
  prepare for next round/1(fOutput) -> Divide5/2
  Switch3/1 -> prepare for next round/1(fOutput_in)  "fOutput"
  IsNaN1/1 -> Switch2/2
  Add/1 -> IsNaN1/1, Switch2/3, Switch3/3
  IsInf1/1 -> Switch3/2
  Switch2/1 -> IsInf1/1
  Constant1/1 -> Switch2/1, Switch3/1
  Divide4/1 -> Add/5
  Divide3/1 -> Add/4
  Divide2/1 -> Add/3
  Divide1/1 -> Add/2
  Divide/1 -> Add/1
  Data Store Read8/1 -> Divide4/1
  Data Store Read7/1 -> Divide4/2
  Data Store Read5/1 -> Divide3/2
  Data Store Read6/1 -> Divide3/1
  Data Store Read4/1 -> Divide2/2
  Data Store Read1/1 -> Divide2/1
  Data Store Read3/1 -> Divide1/2
  Data Store Read/1 -> Divide1/1
  Data Store Read2/1 -> Divide/1
  Switch1/1 -> Divide/2
  IsInf/1 -> Switch1/2
  Switch/1 -> IsInf/1
  Constant/1 -> Switch/1, Switch1/1
  IsNaN/1 -> Switch/2
  fNewInput/1 -> IsNaN/1, Switch/3, Switch1/3, prepare for next round/2(fNewInput)

== system Target_Control_System/Target_Control_System/MainLoop/pitchMotor_mainLoop/mainTask_pitch/motorTaskMainFastStep()/Mechanical System - Pitch/processSensors(&oPitch)/Input (motor) side sensor/updateGbxOutput/updateAngles ==
  fCurrentOutputAngle : Inport
  fNewInputAngle : Inport  Port=2
  Data Store Write : DataStoreWrite  DataStoreName=oPitch  DataStoreElements=oPitch.oMot_.oState_.oPosSensor_.oGbx_.fCurrentOutputAngle_  IndexOptions=Index vector (dialog)  Indices=1  OutputSizes=1
  Data Store Write1 : DataStoreWrite  DataStoreName=oPitch  DataStoreElements=oPitch.oMot_.oState_.oPosSensor_.oGbx_.fPreviousInputAngle_  IndexOptions=Index vector (dialog)  Indices=1  OutputSizes=1
  wires:
  fNewInputAngle/1 -> Data Store Write1/1
  fCurrentOutputAngle/1 -> Data Store Write/1

== system Target_Control_System/Target_Control_System/MainLoop/pitchMotor_mainLoop/mainTask_pitch/motorTaskMainFastStep()/Observer Confidence - Pitch/Automatic switching to sensorless/Switch to sensored? /Switch to sensored/Angle To +-pi ==
  Angle In : Inport
  Add4 : Sum  Inputs=-+
  Add5 : Sum
  Equal4 : RelationalOperator  Operator=>  OutDataTypeStr=boolean  RndMeth=Simplest
  Equal6 : RelationalOperator  Operator=<  OutDataTypeStr=boolean  RndMeth=Simplest
  Pi5 : Constant  Value=pi  OutDataTypeStr=single  SampleTime=-1
  Pi6 : Constant  Value=2*pi  OutDataTypeStr=single  SampleTime=-1
  Pi7 : Constant  Value=-pi  OutDataTypeStr=single  SampleTime=-1
  Pi9 : Constant  Value=2*pi  OutDataTypeStr=single  SampleTime=-1
  Switch : Switch  Criteria=u2 > Threshold
  Switch4 : Switch  Criteria=u2 > Threshold
  Angle Out : Outport
  wires:
  Switch/1 -> Equal6/1, Add5/2, Switch4/3
  Pi7/1 -> Equal6/2
  Add4/1 -> Switch/1
  Pi9/1 -> Add5/1
  Pi5/1 -> Equal4/2
  Equal4/1 -> Switch/2
  Switch4/1 -> Angle Out/1
  Angle In/1 -> Equal4/1, Add4/2, Switch/3
  Add5/1 -> Switch4/1
  Equal6/1 -> Switch4/2
  Pi6/1 -> Add4/1

== system Target_Control_System/Target_Control_System/MainLoop/pitchMotor_mainLoop/mainTask_pitch/motorTaskMainFastStep()/Observer Confidence - Pitch/Automatic switching to sensorless/Switch to sensorless?/Switch to sensorless/Angle To +-pi ==
  Angle In : Inport
  Add4 : Sum  Inputs=-+
  Add5 : Sum
  Equal4 : RelationalOperator  Operator=>  OutDataTypeStr=boolean  RndMeth=Simplest
  Equal6 : RelationalOperator  Operator=<  OutDataTypeStr=boolean  RndMeth=Simplest
  Pi5 : Constant  Value=pi  OutDataTypeStr=single  SampleTime=-1
  Pi6 : Constant  Value=2*pi  OutDataTypeStr=single  SampleTime=-1
  Pi7 : Constant  Value=-pi  OutDataTypeStr=single  SampleTime=-1
  Pi9 : Constant  Value=2*pi  OutDataTypeStr=single  SampleTime=-1
  Switch : Switch  Criteria=u2 > Threshold
  Switch4 : Switch  Criteria=u2 > Threshold
  Angle Out : Outport
  wires:
  Switch/1 -> Equal6/1, Add5/2, Switch4/3
  Pi7/1 -> Equal6/2
  Add4/1 -> Switch/1
  Pi9/1 -> Add5/1
  Pi5/1 -> Equal4/2
  Equal4/1 -> Switch/2
  Switch4/1 -> Angle Out/1
  Angle In/1 -> Equal4/1, Add4/2, Switch/3
  Add5/1 -> Switch4/1
  Equal6/1 -> Switch4/2
  Pi6/1 -> Add4/1

== system Target_Control_System/Target_Control_System/MainLoop/pitchMotor_mainLoop/mainTask_pitch/motorTaskMainFastStep()/Software Overcurrent Protection - Pitch/checkForHwOvercurrents(&oPitch)/gateDriverStatus/IncludeCustomCode/System Update ==

== system Target_Control_System/Target_Control_System/MainLoop/tiltMotor_mainLoop/Decimation gate for 200 Hz Tilt/motorTaskMainDecimationAStep(&oTilt)/Position control checks/Position control mode/Check fighting controllers/Enabled Subsystem/Enabled Subsystem ==
  note: This is the slave inverter
  Enable : EnablePort
  Chart : Stateflow chart  TreatAsAtomicUnit=on

== system Target_Control_System/Target_Control_System/MainLoop/tiltMotor_mainLoop/Decimation gate for 200 Hz Tilt/motorTaskMainDecimationAStep(&oTilt)/Position control checks/Position control mode/checkSensorLimits(&oTilt)/Check broken sensor/All other sensor types ==
  note: All other sensors have a similar interface
  Enable : EnablePort
  Chart : Stateflow chart  TreatAsAtomicUnit=on

== system Target_Control_System/Target_Control_System/MainLoop/tiltMotor_mainLoop/Decimation gate for 200 Hz Tilt/motorTaskMainDecimationAStep(&oTilt)/Position control checks/Position control mode/checkSensorLimits(&oTilt)/Check broken sensor/Resolver ==
  note: This one is somewhat special.
      | The fault code is the 8 bit word coming from the AD2S1210 resolver interface.
      | Some bits are warnigs, some are errors.
      | On ideal hardware the reported code is zero, but we're not quite there yet.
      | From the data sheet:
      |     Table 26. Fault Register Bit Descriptions
      |     Bit  Description
      |     D7   Sine/cosine inputs clipped
      |     D6   Sine/cosine inputs below LOS threshold
      |     D5   Sine/cosine inputs exceed DOS overrange threshold
      |     D4   Sine/cosine inputs exceed DOS mismatch threshold
      |     D3   Tracking error exceeds LOT threshold
      |     D2   Velocity exceeds maximum tracking rate
      |     D1   Phase error exceeds phase lock range
      |     D0   Configuration parity error
      | Understanding in November 2019:
      |     D0-D3 are generally 'true' errors (if set, the result is garbage)
      |     D4-D7 are generally warnings. (often when set, the angle result is actually still valid)
  Enable : EnablePort
  Chart : Stateflow chart  TreatAsAtomicUnit=on

== system Target_Control_System/Target_Control_System/MainLoop/tiltMotor_mainLoop/Decimation gate for 200 Hz Tilt/motorTaskMainDecimationAStep(&oTilt)/Position control checks/Position control mode/checkSensorLimits(&oTilt)/Check delta input-output/Enabled Subsystem ==
  Enable : EnablePort
  Chart : Stateflow chart  TreatAsAtomicUnit=on

== system Target_Control_System/Target_Control_System/MainLoop/tiltMotor_mainLoop/Decimation gate for 200 Hz Tilt/motorTaskMainDecimationAStep(&oTilt)/Position control checks/Position control mode/checkSensorLimits(&oTilt)/Check for stuck sensor/Enabled Subsystem ==
  Enable : EnablePort
  Chart : Stateflow chart  TreatAsAtomicUnit=on

== system Target_Control_System/Target_Control_System/MainLoop/tiltMotor_mainLoop/Decimation gate for 200 Hz Tilt/motorTaskMainDecimationAStep(&oTilt)/Position control checks/Position control mode/checkSensorLimits(&oTilt)/Read sensor flags/nonresolverSensorCodes ==
  Enable : EnablePort
  ModelSource : Subsystem  Variant=on

== system Target_Control_System/Target_Control_System/MainLoop/tiltMotor_mainLoop/Decimation gate for 200 Hz Tilt/motorTaskMainDecimationAStep(&oTilt)/Position control checks/Position control mode/checkSensorLimits(&oTilt)/Read sensor flags/resolverSensorCodes ==
  Enable : EnablePort
  ModelSource : Subsystem  Variant=on

== system Target_Control_System/Target_Control_System/MainLoop/tiltMotor_mainLoop/mainTask_tilt/motorTaskMainFastStep(&oTilt)/Automatic switching to sensorless - Tilt/Automatic switching to sensorless/Switch to sensored /Switch to sensored/Angle To +-pi ==
  Angle In : Inport
  Add4 : Sum  Inputs=-+
  Add5 : Sum
  Equal4 : RelationalOperator  Operator=>  OutDataTypeStr=boolean  RndMeth=Simplest
  Equal6 : RelationalOperator  Operator=<  OutDataTypeStr=boolean  RndMeth=Simplest
  Pi5 : Constant  Value=pi  OutDataTypeStr=single  SampleTime=-1
  Pi6 : Constant  Value=2*pi  OutDataTypeStr=single  SampleTime=-1
  Pi7 : Constant  Value=-pi  OutDataTypeStr=single  SampleTime=-1
  Pi9 : Constant  Value=2*pi  OutDataTypeStr=single  SampleTime=-1
  Switch : Switch  Criteria=u2 > Threshold
  Switch4 : Switch  Criteria=u2 > Threshold
  Angle Out : Outport
  wires:
  Switch/1 -> Equal6/1, Add5/2, Switch4/3
  Pi7/1 -> Equal6/2
  Add4/1 -> Switch/1
  Pi9/1 -> Add5/1
  Pi5/1 -> Equal4/2
  Equal4/1 -> Switch/2
  Switch4/1 -> Angle Out/1
  Angle In/1 -> Equal4/1, Add4/2, Switch/3
  Add5/1 -> Switch4/1
  Equal6/1 -> Switch4/2
  Pi6/1 -> Add4/1

== system Target_Control_System/Target_Control_System/MainLoop/tiltMotor_mainLoop/mainTask_tilt/motorTaskMainFastStep(&oTilt)/Automatic switching to sensorless - Tilt/Automatic switching to sensorless/Switch to sensorless?/Switch to sensorless/Angle To +-pi ==
  Angle In : Inport
  Add4 : Sum  Inputs=-+
  Add5 : Sum
  Equal4 : RelationalOperator  Operator=>  OutDataTypeStr=boolean  RndMeth=Simplest
  Equal6 : RelationalOperator  Operator=<  OutDataTypeStr=boolean  RndMeth=Simplest
  Pi5 : Constant  Value=pi  OutDataTypeStr=single  SampleTime=-1
  Pi6 : Constant  Value=2*pi  OutDataTypeStr=single  SampleTime=-1
  Pi7 : Constant  Value=-pi  OutDataTypeStr=single  SampleTime=-1
  Pi9 : Constant  Value=2*pi  OutDataTypeStr=single  SampleTime=-1
  Switch : Switch  Criteria=u2 > Threshold
  Switch4 : Switch  Criteria=u2 > Threshold
  Angle Out : Outport
  wires:
  Switch/1 -> Equal6/1, Add5/2, Switch4/3
  Pi7/1 -> Equal6/2
  Add4/1 -> Switch/1
  Pi9/1 -> Add5/1
  Pi5/1 -> Equal4/2
  Equal4/1 -> Switch/2
  Switch4/1 -> Angle Out/1
  Angle In/1 -> Equal4/1, Add4/2, Switch/3
  Add5/1 -> Switch4/1
  Equal6/1 -> Switch4/2
  Pi6/1 -> Add4/1

== system Target_Control_System/Target_Control_System/MainLoop/tiltMotor_mainLoop/mainTask_tilt/motorTaskMainFastStep(&oTilt)/Mechanical System - Tilt/processSensors(&oPitch)/Input (motor) side sensor/ /angleClip (+-pi) ==
  Angle_In : Inport
  Add1 : Sum  Inputs=-+
  Add12 : Sum  Inputs=-+
  Add2 : Sum
  Add3 : Sum
  Equal1 : RelationalOperator  Operator=>  OutDataTypeStr=boolean  RndMeth=Simplest
  Equal2 : RelationalOperator  Operator=<  OutDataTypeStr=boolean  RndMeth=Simplest
  Equal3 : RelationalOperator  Operator=<  OutDataTypeStr=boolean  RndMeth=Simplest
  Equal5 : RelationalOperator  Operator=>  OutDataTypeStr=boolean  RndMeth=Simplest
  Pi : Constant  Value=pi  OutDataTypeStr=single  SampleTime=-1
  Pi1 : Constant  Value=2*pi  OutDataTypeStr=single  SampleTime=-1
  Pi2 : Constant  Value=-pi  OutDataTypeStr=single  SampleTime=-1
  Pi3 : Constant  Value=2*pi  OutDataTypeStr=single  SampleTime=-1
  Pi4 : Constant  Value=-pi  OutDataTypeStr=single  SampleTime=-1
  Pi8 : Constant  Value=pi  OutDataTypeStr=single  SampleTime=-1
  Switch{1..3,5} (4 alike) : Switch  Criteria=u2 > Threshold  Threshold=0.5
  Angle_Out : Outport
  wires:
  Switch3/1 -> Switch2/1
  Equal2/1 -> Switch3/2
  Switch5/1 -> Switch2/3, Add3/2, Equal3/1
  Add2/1 -> Switch3/1
  Pi3/1 -> Add3/1, Add2/1
  Add3/1 -> Switch3/3, Equal2/1, Add2/2
  Pi4/1 -> Equal2/2
  Switch2/1 -> Angle_Out/1
  Equal3/1 -> Switch2/2
  Pi2/1 -> Equal3/2
  Switch1/1 -> Switch5/1
  Add1/1 -> Switch1/1
  Equal5/1 -> Switch1/2
  Pi8/1 -> Equal5/2
  Add12/1 -> Equal5/1, Add1/2, Switch1/3
  Pi/1 -> Equal1/2
  Equal1/1 -> Switch5/2
  Angle_In/1 -> Add12/2, Equal1/1, Switch5/3
  Pi1/1 -> Add12/1, Add1/1

== system Target_Control_System/Target_Control_System/MainLoop/tiltMotor_mainLoop/mainTask_tilt/motorTaskMainFastStep(&oTilt)/Mechanical System - Tilt/processSensors(&oPitch)/Input (motor) side sensor/Compute Speed From Sensor/softwareIirFilterStep()1 ==
  fNewInput : Inport
  Add : Sum  Inputs=+++--
  Constant : Constant  Value=0  OutDataTypeStr=single  SampleTime=-1
  Constant1 : Constant  Value=0  OutDataTypeStr=single  SampleTime=-1
  Data Store Read : DataStoreRead  DataStoreName=oTilt  DataStoreElements=oTilt.oMot_.oState_.oPosSensor_.oInputSensorSpeedFilter_.afPreviousInputs_.h0  IndexOptions=Index vector (dialog)  Indices=1  OutputSizes=1
  Data Store Read1 : DataStoreRead  DataStoreName=oTilt  DataStoreElements=oTilt.oMot_.oState_.oPosSensor_.oInputSensorSpeedFilter_.afPreviousInputs_.h1  IndexOptions=Index vector (dialog)  Indices=1  OutputSizes=1
  Data Store Read2 : DataStoreRead  DataStoreName=oTilt  DataStoreElements=oTilt.oMot_.oState_.oPosSensor_.oInputSensorSpeedFilter_.afConstantsB_.h0  IndexOptions=Index vector (dialog)  Indices=1  OutputSizes=1
  Data Store Read3 : DataStoreRead  DataStoreName=oTilt  DataStoreElements=oTilt.oMot_.oState_.oPosSensor_.oInputSensorSpeedFilter_.afConstantsB_.h1  IndexOptions=Index vector (dialog)  Indices=1  OutputSizes=1
  Data Store Read4 : DataStoreRead  DataStoreName=oTilt  DataStoreElements=oTilt.oMot_.oState_.oPosSensor_.oInputSensorSpeedFilter_.afConstantsB_.h2  IndexOptions=Index vector (dialog)  Indices=1  OutputSizes=1
  Data Store Read5 : DataStoreRead  DataStoreName=oTilt  DataStoreElements=oTilt.oMot_.oState_.oPosSensor_.oInputSensorSpeedFilter_.afConstantsA_.h1  IndexOptions=Index vector (dialog)  Indices=1  OutputSizes=1
  Data Store Read6 : DataStoreRead  DataStoreName=oTilt  DataStoreElements=oTilt.oMot_.oState_.oPosSensor_.oInputSensorSpeedFilter_.afPreviousOutputs_.h0  IndexOptions=Index vector (dialog)  Indices=1  OutputSizes=1
  Data Store Read7 : DataStoreRead  DataStoreName=oTilt  DataStoreElements=oTilt.oMot_.oState_.oPosSensor_.oInputSensorSpeedFilter_.afConstantsA_.h2  IndexOptions=Index vector (dialog)  Indices=1  OutputSizes=1
  Data Store Read8 : DataStoreRead  DataStoreName=oTilt  DataStoreElements=oTilt.oMot_.oState_.oPosSensor_.oInputSensorSpeedFilter_.afPreviousOutputs_.h1  IndexOptions=Index vector (dialog)  Indices=1  OutputSizes=1
  Data Store Read9 : DataStoreRead  DataStoreName=oTilt  DataStoreElements=oTilt.oMot_.oState_.oPosSensor_.oInputSensorSpeedFilter_.afConstantsA_.h0  IndexOptions=Index vector (dialog)  Indices=1  OutputSizes=1
  Data Store Write41 : DataStoreWrite  DataStoreName=oTilt  DataStoreElements=oTilt.oMot_.oState_.oPosSensor_.oInputSensorSpeedFilter_.fFilterOutput_  IndexOptions=Index vector (dialog)  Indices=1  OutputSizes=1
  Divide{,1..5} (6 alike) : Product  Inputs=**
  IsInf : RelationalOperator  Operator=isInf  OutDataTypeStr=boolean  RndMeth=Simplest
  IsInf1 : RelationalOperator  Operator=isInf  OutDataTypeStr=boolean  RndMeth=Simplest
  IsNaN : RelationalOperator  Operator=isNaN  OutDataTypeStr=boolean  RndMeth=Simplest
  IsNaN1 : RelationalOperator  Operator=isNaN  OutDataTypeStr=boolean  RndMeth=Simplest
  Switch{,1..3} (4 alike) : Switch  Criteria=u2 > Threshold
  prepare for next round : Subsystem
  fFilterOutput : Outport
  wires:
  Divide1/1 -> Add/2
  Add/1 -> IsNaN1/1, Switch2/3, Switch3/3
  Divide5/1 -> fFilterOutput/1, Data Store Write41/1
  Data Store Read9/1 -> Divide5/1
  prepare for next round/1(fOutput) -> Divide5/2
  Switch3/1 -> prepare for next round/1(fOutput_in)  "fOutput"
  IsNaN1/1 -> Switch2/2
  IsInf1/1 -> Switch3/2
  Switch2/1 -> IsInf1/1
  Constant1/1 -> Switch2/1, Switch3/1
  Divide4/1 -> Add/5
  Divide3/1 -> Add/4
  Divide2/1 -> Add/3
  Divide/1 -> Add/1
  Data Store Read8/1 -> Divide4/1
  Data Store Read7/1 -> Divide4/2
  Data Store Read5/1 -> Divide3/2
  Data Store Read6/1 -> Divide3/1
  Data Store Read4/1 -> Divide2/2
  Data Store Read1/1 -> Divide2/1
  Data Store Read3/1 -> Divide1/2
  Data Store Read/1 -> Divide1/1
  Data Store Read2/1 -> Divide/1
  Switch1/1 -> Divide/2
  IsInf/1 -> Switch1/2
  Switch/1 -> IsInf/1
  Constant/1 -> Switch/1, Switch1/1
  IsNaN/1 -> Switch/2
  fNewInput/1 -> IsNaN/1, Switch/3, Switch1/3, prepare for next round/2(fNewInput)

== system Target_Control_System/Target_Control_System/MainLoop/tiltMotor_mainLoop/mainTask_tilt/motorTaskMainFastStep(&oTilt)/Mechanical System - Tilt/processSensors(&oPitch)/Input (motor) side sensor/PosSensorProcess_altImplementations/If Action Subsystem ==
  In1 : Inport
  Action Port : ActionPort
  Data Store Read1 : DataStoreRead  DataStoreName=oTilt  DataStoreElements=oTilt.oMot_.oParam_.fOneOverSensorPolepairs_  IndexOptions=Index vector (dialog)  Indices=1  OutputSizes=1
  Data Store Read19 : DataStoreRead  DataStoreName=oTilt  DataStoreElements=oTilt.oMot_.oParam_.fPolePairs_  IndexOptions=Index vector (dialog)  Indices=1  OutputSizes=1
  Product1 : Product  Inputs=3
  Out1 : Outport
  wires:
  Data Store Read1/1 -> Product1/3
  Data Store Read19/1 -> Product1/2
  Product1/1 -> Out1/1
  In1/1 -> Product1/1
